simulink model "bustest2"  (R2018a)
settings: Solver=VariableStepAuto  StartTime=0.0  StopTime=10.0  RelTol=1e-3
undefined symbols (not defined in the file or in its folder): BandWidth, BaseVoltage, CogenEnabled, ControlledTransformerConnection, ControlledTransformerPowers, ControlledTransformerVoltages, ILDC, IsReversible, LDC_Z, m, MaxTap, MinTap, n, PTratio, RevBand, RevDelay, RevPowerThreshold, RevVreg, TapDelay, TapIncrement, TapLimitPerChange, TapWinding, UsingRegulatedBus, Vlimit, Vreg, VTerminal
settings Model: Creator=Michael Girbino  LastModifiedBy=Michael Girbino
settings CodeAppCC: StateflowObjectComments=on

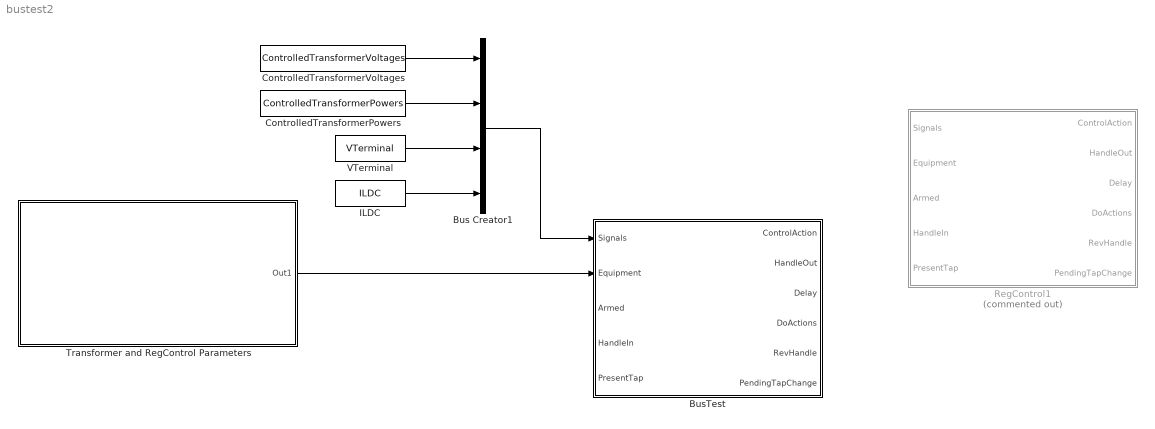
== system bustest2 ==
  Bus Creator1 : BusCreator  Inputs=4  OutDataTypeStr=Bus: SignalBus
  BusTest : Stateflow chart  TreatAsAtomicUnit=on
  ControlledTransformerPowers : Constant  Value=ControlledTransformerPowers
  ControlledTransformerVoltages : Constant  Value=ControlledTransformerVoltages
  ILDC : Constant  Value=ILDC
  RegControl1 : Stateflow chart  Commented=on  TreatAsAtomicUnit=on
  Transformer and RegControl Parameters : Subsystem
  VTerminal : Constant  Value=VTerminal
  wires:
  ControlledTransformerVoltages/1 -> Bus Creator1/1
  ControlledTransformerPowers/1 -> Bus Creator1/2
  Bus Creator1/1 -> BusTest/1(Signals)
  VTerminal/1 -> Bus Creator1/3
  ILDC/1 -> Bus Creator1/4
  Transformer and RegControl Parameters/1(Out1) -> BusTest/2(Equipment)

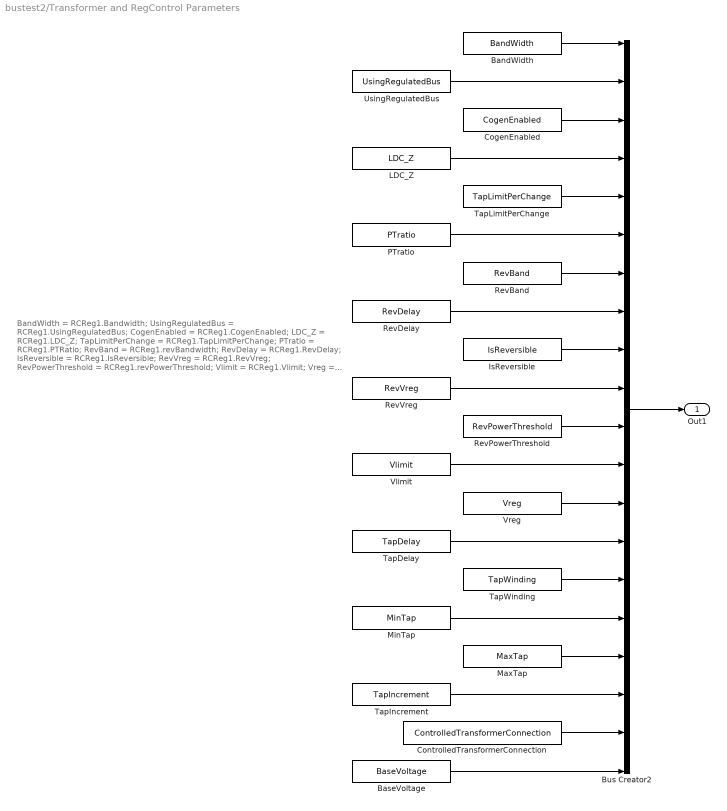
== system bustest2/Transformer and RegControl Parameters ==
  note: BandWidth = RCReg1.Bandwidth;
      | UsingRegulatedBus = RCReg1.UsingRegulatedBus;
      | CogenEnabled = RCReg1.CogenEnabled;
      | LDC_Z = RCReg1.LDC_Z;
      | TapLimitPerChange = RCReg1.TapLimitPerChange;
      | PTratio = RCReg1.PTRatio;
      | RevBand = RCReg1.revBandwidth;
      | RevDelay = RCReg1.RevDelay;
      | IsReversible = RCReg1.IsReversible;
      | RevVreg = RCReg1.RevVreg;
      | RevPowerThreshold = RCReg1.revPowerThreshold;
      | Vlimit = RCReg1.Vlimit;
      | Vreg = RCReg1.Vreg;
      | TapDelay = RCReg1.TapDelay;
      | TapWinding = RCReg1.xsfWinding;
      |
      | % PresentTap = Equipment.TReg1.Winding(TapWinding).puTap;
      | MinTap = TReg1.Winding(TapWinding).MinTap;
      | MaxTap = TReg1.Winding(TapWinding).MaxTap;
      | TapIncrement = TReg1.Winding(TapWinding).TapIncrement;
      | ControlledTransformerConnection = TReg1.Winding(TapWinding).Connection;
      | BaseVoltage = TReg1.Winding(TapWinding).Vbase;
  BandWidth : Constant  Value=BandWidth
  BaseVoltage : Constant  Value=BaseVoltage
  Bus Creator2 : BusCreator  Inputs=20  OutDataTypeStr=Bus: EquipmentBus
  CogenEnabled : Constant  Value=CogenEnabled
  ControlledTransformerConnection : Constant  Value=ControlledTransformerConnection
  IsReversible : Constant  Value=IsReversible
  LDC_Z : Constant  Value=LDC_Z
  MaxTap : Constant  Value=MaxTap
  MinTap : Constant  Value=MinTap
  PTratio : Constant  Value=PTratio
  RevBand : Constant  Value=RevBand
  RevDelay : Constant  Value=RevDelay
  RevPowerThreshold : Constant  Value=RevPowerThreshold
  RevVreg : Constant  Value=RevVreg
  TapDelay : Constant  Value=TapDelay
  TapIncrement : Constant  Value=TapIncrement
  TapLimitPerChange : Constant  Value=TapLimitPerChange
  TapWinding : Constant  Value=TapWinding
  UsingRegulatedBus : Constant  Value=UsingRegulatedBus
  Vlimit : Constant  Value=Vlimit
  Vreg : Constant  Value=Vreg
  Out1 : Outport
  wires:
  TapIncrement/1 -> Bus Creator2/18
  UsingRegulatedBus/1 -> Bus Creator2/2
  BandWidth/1 -> Bus Creator2/1
  BaseVoltage/1 -> Bus Creator2/20
  ControlledTransformerConnection/1 -> Bus Creator2/19
  MaxTap/1 -> Bus Creator2/17
  MinTap/1 -> Bus Creator2/16
  TapWinding/1 -> Bus Creator2/15
  TapDelay/1 -> Bus Creator2/14
  Vreg/1 -> Bus Creator2/13
  Vlimit/1 -> Bus Creator2/12
  RevPowerThreshold/1 -> Bus Creator2/11
  RevVreg/1 -> Bus Creator2/10
  IsReversible/1 -> Bus Creator2/9
  RevDelay/1 -> Bus Creator2/8
  RevBand/1 -> Bus Creator2/7
  PTratio/1 -> Bus Creator2/6
  TapLimitPerChange/1 -> Bus Creator2/5
  LDC_Z/1 -> Bus Creator2/4
  CogenEnabled/1 -> Bus Creator2/3
  Bus Creator2/1 -> Out1/1

== stateflow chart bustest2/RegControl1 ==
  settings: executeAtInitialization=1
  state ControlFlow
    state DetermineReversePendingLookingForward
      state CorrectFalseReversePending
        (default) -> (junction 108)
        (junction 108) -> (junction 109) [order 1] : [FwdPower < (-1*RevPowerThreshold)]
        (junction 108) -> (junction 111) [order 2]
        (junction 109) -> (junction 112) : {ReversePending = true;
            | RevHandle = ...
            | Push(ActionCodes.ACTION_REVERSE, ...
            | RevDelay);
            | }
        (junction 112) -> (junction 111)
      state CorrectTrueReversePending
        (default) -> (junction 804)
        (junction 804) -> (junction 123) [order 1] : [FwdPower >= (-1*RevPowerThreshold)]
        (junction 804) -> (junction 809) [order 2]
        (junction 123) -> (junction 806) : % Reset ReversePending:
            | % Delete RevHandle from ControlQueue
            | {DoActions.data = QueueActions.DELETE;
            | send(DoActions);
            | ReversePending = false;
            | RevHandle = 0;}
        (junction 806) -> (junction 809)
      state Finished
        en: GET_VOLTAGE = true;
      (default) -> (junction 106) : {FwdPower = -1*real( ControlledTransformerPower(ElementTerminal) );}
          | % Should we reverse?
      (junction 106) -> ControlFlow.DetermineReversePendingLookingForward.CorrectFalseReversePending [order 1] : [~ReversePending]
      (junction 106) -> (junction 110) [order 2]
      ControlFlow.DetermineReversePendingLookingForward.CorrectFalseReversePending -> (junction 110)
      (junction 110) -> (junction 120)
      (junction 120) -> ControlFlow.DetermineReversePendingLookingForward.CorrectTrueReversePending [order 1] : [ReversePending]
      (junction 120) -> (junction 122) [order 2]
      ControlFlow.DetermineReversePendingLookingForward.CorrectTrueReversePending -> (junction 122)
      (junction 122) -> ControlFlow.DetermineReversePendingLookingForward.Finished
    state DetermineReversePendingLookingReverseOrCogen
      state CorrectFalseReversePending
        (default) -> (junction 130)
        (junction 130) -> (junction 138) [order 1] : [FwdPower > RevPowerThreshold]
        (junction 130) -> (junction 137) [order 2]
        (junction 138) -> (junction 136) : {ReversePending = true;
            | RevHandle = ...
            | Push(ActionCodes.ACTION_REVERSE, ...
            | RevDelay);
            | }
        (junction 136) -> (junction 137)
      state CorrectTrueReversePending
        (default) -> (junction 154)
        (junction 154) -> (junction 799) [order 1] : [FwdPower <= RevPowerThreshold]
        (junction 154) -> (junction 792) [order 2]
        (junction 799) -> (junction 148) : % Reset ReversePending:
            | {ReversePending = false;}
        (junction 148) -> (junction 792)
      state Finished
        en: REV_NEUTRAL = true;
      (default) -> (junction 144) : {FwdPower = -1*real( ControlledTransformerPower(ElementTerminal) );}
          | % If reversed, check if power is back in forward direction
      (junction 144) -> ControlFlow.DetermineReversePendingLookingReverseOrCogen.CorrectFalseReversePending [order 1] : [~ReversePending]
      (junction 144) -> (junction 139) [order 2]
      ControlFlow.DetermineReversePendingLookingReverseOrCogen.CorrectFalseReversePending -> (junction 139)
      (junction 139) -> (junction 147)
      (junction 147) -> ControlFlow.DetermineReversePendingLookingReverseOrCogen.CorrectTrueReversePending [order 1] : [ReversePending]
      (junction 147) -> (junction 151) [order 2]
      ControlFlow.DetermineReversePendingLookingReverseOrCogen.CorrectTrueReversePending -> (junction 151)
      (junction 151) -> ControlFlow.DetermineReversePendingLookingReverseOrCogen.Finished
    state ReverseNeutralCase
      state Finished
        send(GET_VOLTAGE);
      state Exiting
        en: EXIT = true;
      (default) -> (junction 166)
      (junction 166) -> (junction 155) [order 1] : % tap change not specified as needed:
          | [~Armed]
      (junction 166) -> ControlFlow.ReverseNeutralCase.Finished [order 2]
      (junction 155) -> (junction 160) : {PendingTapChange = 0.0;}
      (junction 160) -> (junction 167) [order 1] : [abs(PresentTap - 1.0) < EPSILON]
      (junction 160) -> Exiting [order 2]
      (junction 167) -> (junction 518) : %{Increment = TapIncrement(TapWinding);
          | %PendingTapChange = round( (1.0 - ...
          | %PresentTap(TapWinding)) / Increment ) * Increment;}
          | {PendingTapChange = ...
          | round( (1.0 - TapWinding) / TapIncrement ) * TapIncrement;}
      (junction 518) -> (junction 519) [order 1] : [PendingTapChange ~= 0.0 && ~Armed]
      (junction 519) -> (junction 521) : {% Push ACTION_TAPCHANGE
          | % to ControlQueue with TapDelay:
          | Push(ActionCodes.ACTION_TAPCHANGE, TapDelay);
          | Armed = true;}
      (junction 518) -> (junction 520) [order 2]
      (junction 521) -> (junction 520)
      (junction 520) -> (junction 164)
      (junction 164) -> Exiting
    state GetVoltage
      state Finished
        en: DETERMINE_VLOCALBUS = true;
      (default) -> (junction 75)
      (junction 75) -> (junction 76) [order 1] : [UsingRegulatedBus]
      (junction 75) -> ControlFlow.GetVoltage.Finished [order 2] : {VBuffer = ControlledTransformerWindingVoltages;
          | %ControlledTransformer.GetWindingVoltages;
          | Vcontrol = GetControlVoltage;}
      (junction 76) -> (junction 78) : {TransformerConnection = ControlledTransformerConnection;
          | %TransformerConnection = ControlledTransformer.Winding(ElementTerminal).Connection;
          | %Vterminal = ComputeVTerminal;
          | }
      (junction 78) -> ControlFlow.GetVoltage.Finished
    state DetermineVlocalbus
      state Finished
        en: GET_VOLTAGEWLDC = true;
      (default) -> (junction 321)
      (junction 321) -> (junction 322) [order 1] : % Voltage limit for bus connected to regulated winding; default = 0.0 (inactive)
          | [VlimitActive]
      (junction 321) -> ControlFlow.DetermineVlocalbus.Finished [order 2] : {Vlocalbus = 0.0;}
      (junction 322) -> (junction 332)
      (junction 332) -> (junction 333) [order 1] : % when controlled transformer is different from LDC PTransformer
          | [UsingRegulatedBus]
      (junction 332) -> (junction 334) [order 2] : % controlled transformer is
          | % the LDC PTransformer
          | {Vlocalbus = abs(Vcontrol);}
      (junction 333) -> (junction 335) : {%ControlledTransformer.GetWindingVoltages(ElementTerminal, VBuffer);
          | Vlocalbus = abs( VBuffer(1) / PTRatio );}
      (junction 335) -> (junction 334)
      (junction 334) -> (junction 324)
      (junction 324) -> ControlFlow.DetermineVlocalbus.Finished
    state GetVoltageWithLDC
      state RX_LDCmode
        (default) -> (junction 365)
        (junction 365) -> (junction 366) [order 1] : [InReverseMode || InCogenMode]
        (junction 365) -> (junction 367) [order 2] : {VLDC = complex(R, X) * complex( real(ILDC), imag(ILDC) );}
        (junction 366) -> (junction 368) : {VLDC = complex(revR, revX) * complex( real(ILDC), imag(ILDC) );}
        (junction 368) -> (junction 367)
      state Z_LDCmode
        (default) -> (junction 387)
        (junction 387) -> (junction 388) [order 1] : [InReverseMode || InCogenMode]
        (junction 387) -> (junction 389) [order 2] : {Vcontrol = abs(Vcontrol) - abs(ILDC) * LDC_Z;}
        (junction 388) -> (junction 390) : {Vcontrol = abs(Vcontrol) - abs(ILDC) * revLDC_Z;}
        (junction 390) -> (junction 389)
      state Finished
        en: GET_TEST_VALUES = true;
      (default) -> (junction 354) : %{%%ControlledElement.GetCurrents(CBuffer);
          | %%Convert current to control current by CTRating:
          | %ILDC = ControlledElementCurrents( ControlledElementNconds * (ElementTerminal - 1) + ControlledPhase);}
      (junction 354) -> RX_LDCmode [order 1] : % Standard R, X LDC
          | [LDC_Z == 0.0]
      (junction 354) -> Z_LDCmode [order 2] : % Beckwith LDC_Z control mode
      Z_LDCmode -> ControlFlow.GetVoltageWithLDC.Finished
      RX_LDCmode -> ControlFlow.GetVoltageWithLDC.Finished
    state GetTestValues
      state Finished
        en:
        DETERMINE_TAP_CHANGE = true;
      (default) -> (junction 398) : % assumes looking forward:
          | {Vactual = abs(Vcontrol);}
      (junction 398) -> (junction 399) [order 1] : [InReverseMode]
      (junction 398) -> ControlFlow.GetTestValues.Finished [order 2] : {VregTest = Vreg;
          | BandTest = Bandwidth;}
      (junction 399) -> (junction 401) : {Vactual = Vactual / PresentTap;
          | VregTest = RevVreg;
          | BandTest = RevBandwidth;}
      (junction 401) -> ControlFlow.GetTestValues.Finished
    state DetermineTapChangeIsNeeded
      state Finished
        en:
        MAKE_TAP_CHANGE = true;
      (default) -> (junction 409)
      (junction 409) -> (junction 410) [order 1] : % difference between desired and actual > half bandwidth
          | [abs(VregTest - Vactual) > BandTest/2.0]
      (junction 409) -> ControlFlow.DetermineTapChangeIsNeeded.Finished [order 2] : {TapChangeIsNeeded = false;}
      (junction 410) -> (junction 412) : {TapChangeIsNeeded = true;}
      (junction 412) -> ControlFlow.DetermineTapChangeIsNeeded.Finished
    state MakeTapChange
      state GetVboostFromVlimit
        (default) -> (junction 441)
        (junction 441) -> (junction 446) [order 1] : [Vlocalbus > Vlimit]
        (junction 441) -> (junction 443) [order 2]
        (junction 446) -> (junction 445) : {Vboost = Vlimit - Vlocalbus;}
        (junction 445) -> (junction 443)
      state TapChangeUp
        (default) -> (junction 475)
        (junction 475) -> (junction 476) [order 1] : [PresentTap < MaxTap]
        (junction 475) -> (junction 477) [order 2]
        (junction 476) -> (junction 478) : {% push ACTION_TAPCHANGE to ControlQueue
            | % with delay ComputeTimeDelay(Vactual):
            | Push(ActionCodes.ACTION_TAPCHANGE, ...
            | ComputeTimeDelay(Vactual));
            | Armed = true;}
        (junction 478) -> (junction 477)
      state TapChangeDown
        (default) -> (junction 488) : % going down:
        (junction 488) -> (junction 489) [order 1] : [PresentTap > MinTap]
        (junction 488) -> (junction 490) [order 2]
        (junction 489) -> (junction 491) : {% push ACTION_TAPCHANGE to ControlQueue
            | % with delay ComputeTimeDelay(Vactual):
            | Push(ActionCodes.ACTION_TAPCHANGE, ...
            | ComputeTimeDelay(Vactual));
            | Armed = true;}
        (junction 491) -> (junction 490)
      state Finished
        en: FINISHED = true;
      (default) -> (junction 431) : % compute tapchange:
          | {Vboost = VregTest - Vactual;}
      (junction 431) -> (junction 432) [order 1] : [VlimitActive]
      (junction 431) -> (junction 433) [order 2]
      (junction 432) -> GetVboostFromVlimit
      GetVboostFromVlimit -> (junction 434)
      (junction 434) -> (junction 433)
      (junction 433) -> (junction 435) : {% PU winding boost needed:
          | BoostNeeded = Vboost * PTRatio / BaseVoltage;
          | Increment = TapIncrement(TapWinding);
          | % quantize to an increment:
          | PendingTapChange = round(BoostNeeded/Increment)*Increment;}
      (junction 435) -> (junction 453) : % send initial tap change message to ControlQueue, add delay time to solution control queue:
      (junction 453) -> (junction 454) [order 1] : % only changes 1 tap at a time:
          | [PendingTapChange ~= 0.0 && ~Armed]
      (junction 453) -> ControlFlow.MakeTapChange.Finished [order 2]
      (junction 454) -> (junction 464) : % see of any tap change is possible in desired direction (not saturated):
      (junction 464) -> TapChangeUp [order 1] : % going up:
          | [PendingTapChange > 0.0]
      (junction 464) -> TapChangeDown [order 2]
      TapChangeUp -> (junction 467)
      TapChangeDown -> (junction 466)
      (junction 467) -> (junction 466)
      (junction 466) -> (junction 456)
      (junction 456) -> ControlFlow.MakeTapChange.Finished
    state Finished
    (default) -> (junction 207) : {AssignInputsToLocals();
        | ResetTransitionFlags();}
    (junction 207) -> (junction 208) [order 2]
    (junction 208) -> (junction 86)
    (junction 207) -> (junction 529) [order 1] : [TapLimitPerChange == 0]
    (junction 86) -> (junction 87) [order 1] : [~UsingRegulatedBus]
    (junction 87) -> (junction 61)
    (junction 86) -> (junction 88) [order 2]
    (junction 61) -> (junction 62) [order 1] : [IsReversible || CogenEnabled]
    (junction 61) -> (junction 65) [order 2]
    (junction 62) -> (junction 63)
    (junction 63) -> DetermineReversePendingLookingForward [order 1] : [LookingForward && ~InCogenMode]
    (junction 63) -> DetermineReversePendingLookingReverseOrCogen [order 2]
    DetermineReversePendingLookingForward -> (junction 67) : [GET_VOLTAGE]
    DetermineReversePendingLookingReverseOrCogen -> (junction 175) : [REV_NEUTRAL]
    (junction 175) -> ReverseNeutralCase [order 1] : % mode for which tap change may be executed,
        | % but no reversal made:
        | [ReverseNeutral]
    (junction 175) -> (junction 174) [order 2]
    ReverseNeutralCase -> (junction 174) [order 2] : GET_VOLTAGE
    (junction 174) -> (junction 127)
    ReverseNeutralCase -> (junction 532) [order 1] : [EXIT]
    (junction 65) -> (junction 88)
    (junction 127) -> (junction 65)
    (junction 67) -> (junction 127)
    (junction 88) -> GetVoltage
    (junction 532) -> (junction 529)
    (junction 529) -> (junction 212)
    GetVoltage -> DetermineVlocalbus : [DETERMINE_VLOCALBUS]
    DetermineVlocalbus -> (junction 343) : [GET_VOLTAGEWLDC]
    (junction 343) -> GetVoltageWithLDC [order 1] : % line drop compensation, but not using regulated bus
        | [~UsingRegulatedBus && LDCActive]
    (junction 343) -> (junction 345) [order 2]
    GetVoltageWithLDC -> (junction 346) : [GET_TEST_VALUES]
    (junction 346) -> (junction 345)
    (junction 345) -> GetTestValues
    GetTestValues -> DetermineTapChangeIsNeeded : [DETERMINE_TAP_CHANGE]
    DetermineTapChangeIsNeeded -> (junction 420) : [MAKE_TAP_CHANGE]
    (junction 420) -> MakeTapChange [order 1] : [TapChangeIsNeeded]
    (junction 420) -> (junction 422) [order 2]
    MakeTapChange -> (junction 423) : [FINISHED]
    (junction 423) -> (junction 422)
    (junction 422) -> ControlFlow.Finished
    (junction 212) -> ControlFlow.Finished : {PendingTapChange = 0;}
  state h = Push(CodeVal, DelayVal) [function]
    (default) -> (junction 860) : {ActionCode = CodeVal;
        | Delay = DelayVal;
        | HandleOut = HandleOut + 1;
        | DoActions.data = QueueActions.PUSH;
        | send(DoActions);
        | h = HandleOut;}
  state AssignInputsToLocals [function]
    (default) -> (junction 987) : {BandWidth = Equipment.RCReg1.Bandwidth;
        | UsingRegulatedBus = Equipment.RCReg1.UsingRegulatedBus;
        | CogenEnabled = Equipment.RCReg1.CogenEnabled;
        | LDC_Z = Equipment.RCReg1.LDC_Z;
        | TapLimitPerChange = Equipment.RCReg1.TapLimitPerChange;
        | PTratio = Equipment.RCReg1.PTRatio;
        | RevBand = Equipment.RCReg1.revBandwidth;
        | RevDelay = Equipment.RCReg1.RevDelay;
        | IsReversible = Equipment.RCReg1.IsReversible;
        | RevVreg = Equipment.RCReg1.RevVreg;
        | RevPowerThreshold = Equipment.RCReg1.revPowerThreshold;
        | Vlimit = Equipment.RCReg1.Vlimit;
        | Vreg = Equipment.RCReg1.Vreg;
        | TapDelay = Equipment.RCReg1.TapDelay;
        | TapWinding = Equipment.RCReg1.xsfWinding;
        |
        | % PresentTap = Equipment.TReg1.Winding(TapWinding).puTap;
        | MinTap = Equipment.TReg1.Winding(TapWinding).MinTap;
        | MaxTap = Equipment.TReg1.Winding(TapWinding).MaxTap;
        | TapIncrement = Equipment.TReg1.Winding(TapWinding).TapIncrement;
        | ControlledTransformerConnection = Equipment.TReg1.Winding(TapWinding).Connection;
        | BaseVoltage = Equipment.TReg1.Winding(TapWinding).Vbase;
        |
        | ControlledTransformerWindingVoltages = Signals.ControlledTransformerWindingVoltages;
        | ControlledTransformerPower = Signals.ControlledTransformerPower;
        | VTerminal = Signals.VTerminal;
        | ILDC = Signals.ILDC;
        |
        | VBuffer = zeros(length(ControlledTransformerWindingVoltages));
        | }
    (junction 987) -> (junction 996) [order 1] : [Equipment.RCReg1.R~=0 || Equipment.RCReg1.X~=0 || Equipment.RCReg1.LDC_Z>0]
    (junction 987) -> (junction 991) [order 2] : {LDCActive = false;}
    (junction 996) -> (junction 990) : {LDCActive = true;}
    (junction 990) -> (junction 991)
    (junction 991) -> (junction 722)
    (junction 722) -> (junction 897) [order 1] : [HandleIn > HandleOut]
    (junction 722) -> (junction 898) [order 2]
    (junction 897) -> (junction 899) : {HandleOut = HandleIn;}
    (junction 899) -> (junction 898)
    (junction 898) -> (junction 900)
  note: BandWidth
      | UsingRegulatedBus
      | CogenEnabled
      | LDC_Z
      | TapLimitPerChange
      | PTratio
      | RevBand
      | IsReversible
      | RevVreg
      | Vlimit
      | Vreg
      | ILDC
      | FwdPower
  state ResetTransitionFlags [function]
    (default) -> (junction 886) : {DETERMINE_TAP_CHANGE = false;
        | DETERMINE_VLOCALBUS = false;
        | EXIT = false;
        | FINISHED = false;
        | GET_TEST_VALUES = false;
        | GET_VOLTAGE = false;
        | GET_VOLTAGEWLDC = false;
        | MAKE_TAP_CHANGE = false;
        | REV_NEUTRAL = false;}
  state UpdateControlledTransformerWV [function] [commented out]
    note: Retrieves new value for ControlledTransformerWindingVoltages. Update since last call of AssignInputsToLocals. Necessary because the control flow requires multiple updates to this quantity.
    (default) -> (junction 905) [commented out] : {ControlledTransformerWindingVoltages = ...
        | Inputs.ControlledTransformerWindingVoltages;}
  state UpdateControlledTransformerPower [function] [commented out]
    note: Retrieves new value for ControlledTransformerPower. Update since last call of AssignInputsToLocals. Necessary because the control flow requires multiple updates to this quantity.
    (default) -> (junction 902) [commented out] : {ControlledTransformerPower = ...
        | Inputs.ControlledTransformerPower;}
  state vt = ComputeVTerminal [function] [commented out]
    (default) -> (junction 309) [commented out] : % Iteration through order of admittance matrix
        | % (inherited from CktElement)
    (junction 310) -> (junction 308) [commented out] : [ii <= Yorder]
    (junction 308) -> (junction 311) [commented out] : {vt(ii) = NodeV(NodeRef(ii));}
    (junction 309) -> (junction 310) [commented out] : {ii = 1;}
    (junction 311) -> (junction 310) [commented out] : {ii = ii + 1;}
    (junction 310) -> (junction 312) [commented out]
  state WindingVoltages = GetWindingVoltages(Transformer, IndicatedWinding) [function] [commented out]
    note: Intend to store WindingVoltages in VBuffer.
        | Fills array with voltages across indicated winding
    note: For Delta connections or Line-Line voltages
    (default) -> (junction 969) [commented out] : % Determine whether winding exists
    (junction 923) -> (junction 921) [commented out] : [ii <= Yorder]
    (junction 921) -> (junction 924) [commented out] : {Vterminal(ii) = NodeV( NodeRef(i) );}
    (junction 969) -> (junction 922) [commented out] : [IndicatedWinding >= 1 && IndicatedWinding <= NumWindings]
    (junction 969) -> (junction 971) [commented out]
    (junction 922) -> (junction 923) [commented out] : {ii = 1;}
    (junction 924) -> (junction 923) [commented out] : {ii = ii + 1;}
    (junction 923) -> (junction 925) [commented out] : {k = (IndicatedWinding - 1) * Fnconds;
        | NeutTerm = Fnphases + k + 1;}
    (junction 925) -> (junction 935) [commented out] : {ii = 1;}
    (junction 935) -> (junction 933) [commented out] : [ii <= Fnphases]
    (junction 933) -> (junction 952) [commented out]
    (junction 952) -> (junction 953) [commented out] : [Winding(IndicatedWinding).Connection == Connections.WYE]
    (junction 952) -> (junction 956) [commented out]
    (junction 953) -> (junction 954) [commented out] : {VBuffer(ii) = Vterminal(ii + k) - Vterminal(NeutTerm);}
    (junction 954) -> (junction 955) [commented out]
    (junction 955) -> (junction 959) [commented out]
    (junction 956) -> (junction 957) [commented out] : [Winding(IndicatedWinding).Connection == Connections.DELTA]
    (junction 956) -> (junction 960) [commented out]
    (junction 957) -> (junction 958) [commented out] : {iii = RotatePhases(ii);
        | VBuffer(ii) = ...
        | Vterminal(ii + k) - ...
        | Vterminal(iii+k);}
    (junction 936) -> (junction 935) [commented out] : {ii = ii + 1;}
    (junction 935) -> (junction 937) [commented out] : {WindingVoltages = VBuffer;}
    (junction 958) -> (junction 959) [commented out]
    (junction 959) -> (junction 961) [commented out]
    (junction 961) -> (junction 960) [commented out]
    (junction 960) -> (junction 936) [commented out]
    (junction 937) -> (junction 971) [commented out]
    (junction 971) -> (junction 973) [commented out]
  state Result = GetControlVoltage [function]
    (default) -> (junction 236)
    (junction 236) -> (junction 237) [order 1] : [FPTphase == FPTphases.MAXPHASE]
        | % controlled phase is that with greatest |V|
    (junction 236) -> (junction 240) [order 2]
    (junction 237) -> (junction 260) : {ControlledPhase = 1;
        | % abs is equivalent to Cabs:
        | V = abs( VBuffer(ControlledPhase) );}
        | % Iteration through remaining phases:
    (junction 261) -> (junction 259) [order 1] : [ii <= Nphs]
    (junction 259) -> (junction 270)
    (junction 260) -> (junction 261) : {ii = 2;}
    (junction 270) -> (junction 271) [order 1] : [abs( VBuffer(ControlledPhase)) > V]
        | % if it's GREATER, make it the new V
    (junction 270) -> (junction 272) [order 2]
    (junction 271) -> (junction 273) : {V = VBuffer(ControlledPhase);
        | ControlledPhase = ii;}
    (junction 262) -> (junction 261) : {ii = ii+1;}
    (junction 261) -> (junction 238) [order 2]
    (junction 273) -> (junction 272)
    (junction 272) -> (junction 262) : {Result = VBuffer(FPTphase) / PTRatio;
        | % Complex divided by real
        | }
    (junction 238) -> (junction 239)
    (junction 239) -> (junction 243)
    (junction 240) -> (junction 241) [order 1] : [FPTphase == FPTphases.MINPHASE]
        | % controlled phase is that with least |V|
    (junction 241) -> (junction 282) : {ControlledPhase = 1;
        | % abs is equivalent to Cabs:
        | V = abs( VBuffer(ControlledPhase) );}
        | % Iteration through remaining phases:
    (junction 240) -> (junction 244) [order 2] : % just use one phase because
        | % that's what most controls do:
        | {Result = VBuffer(ControlledPhase) / PTRatio;
        | ControlledPhase = FPTphase;}
    (junction 278) -> (junction 277) [order 1] : [ii <= Nphs]
    (junction 277) -> (junction 291)
    (junction 282) -> (junction 278) : {ii = 2;}
    (junction 291) -> (junction 292) [order 1] : [abs( VBuffer(ControlledPhase)) < V]
        | % if it's LESS, make it the new V
    (junction 291) -> (junction 293) [order 2]
    (junction 292) -> (junction 294) : {V = VBuffer(ControlledPhase);
        | ControlledPhase = ii;}
    (junction 280) -> (junction 278) : {ii = ii+1;}
    (junction 278) -> (junction 242) [order 2]
    (junction 294) -> (junction 293)
    (junction 293) -> (junction 280) : {Result = VBuffer(FPTphase) / PTRatio;
        | % Complex divided by real
        | }
    (junction 242) -> (junction 243)
    (junction 243) -> (junction 245)
    (junction 245) -> (junction 244)
    (junction 244) -> (junction 246)
  state Result = ComputeTimeDelay(Vavg) [function]
    (default) -> (junction 507)
    (junction 507) -> (junction 508) [order 1] : [Finversetime]
    (junction 507) -> (junction 509) [order 2] : % determines which regulator control will act first,
        | % default is 15s
        | {Result = TimeDelay;}
    (junction 508) -> (junction 510) : % TimeDelay is adjusted inversely proportional to
        | % the amount that voltage is outside the band,
        | % down to 10 percent of specified time delay
        | % (Further out of band = band - 1> less time delay)
        | {Result = TimeDelay / min(10.0, 2.0*abs(Vreg - Vavg)/Bandwidth);}
    (junction 510) -> (junction 509)
    (junction 509) -> (junction 511)
  (default) -> ControlFlow
  data: CodeVal function_input; DelayVal function_input; h function_output; vt function_output; IndicatedPhase function_input; RotatedPhase function_output; Transformer function_input; IndicatedWinding function_input; WindingVoltages function_output; Result function_output; Vavg function_input; Result function_output; Signals input Bus: SignalBus; Equipment input Bus: EquipmentBus; BandTest local double =0; BoostNeeded local double =0; Increment local double =0; ReversePending local boolean =false; TapChangeIsNeeded local boolean =false; Vactual local double =0; Vboost local double =0; Vcontrol local double =0; Vlocalbus local double =0; VregTest local double =0; EPSILON local double =1.0e-12; R local double =0; X local double =0; BaseVoltage local double; ControlledPhase local uint8; ElementTerminal local uint8 =1; InCogenMode local boolean =false; InReverseMode local boolean =false; LDCActive local boolean =false; LookingForward local boolean =false; MaxTap local uint8; MinTap local uint8; NodeV local double; RevPowerThreshold local double; ReverseNeutral local boolean =false; TapIncrement local double; TapWinding local uint8 =1; VBuffer local double; VlimitActive local boolean =false; revLDC_Z local double =0; revR local double =0; revX local double =0; TransformerConnection local int32 =0; VLDC local double =0; Vterminal local double; Bandwidth local double =3; CogenEnabled local boolean =false; FwdPower local double =0; ILDC local double =0; IsReversible local boolean =false; LDC_Z local double =0; PTRatio local double =60; RevBandwidth local double =3; RevVreg local double =120; TapLimitPerChange local uint8 =16; UsingRegulatedBus local boolean =false; Vlimit local double =0; Vreg local double =120; ControlAction output Enum: ActionCodes; Armed input boolean =false; HandleOut output double =0; Delay output double =0; DoActions output Enum: QueueActions; RevBackHandle local uint8 =0; RevHandle output uint8 =0; REV_NEUTRAL local boolean =false; RevDelay local double; ControlledTransformerWindingVoltages local double; ControlledTransformerConnection local Enum: Connections; EXIT local boolean =false; FINISHED local boolean =false; GET_TEST_VALUES local boolean =false; MAKE_TAP_CHANGE local boolean =false; DETERMINE_TAP_CHANGE local boolean =false; GET_VOLTAGE local boolean =false; GET_VOLTAGEWLDC local boolean =false; DETERMINE_VLOCALBUS local boolean =false; TapDelay local double; HandleIn input double; PendingTapChange output double; PresentTap input double; ControlledElementCurrents local double; ControlledElementNconds local double; ControlledTransformerPower local double
  function RotatedPhase = RotatePhases(IndicatedPhase):
    | function RotatedPhase = RotatePhases(IndicatedPhase)
    |     HVLeadsLV = false;
    |     % FIRST NEED TO DETERMINE DELTADIRECTION:
    |     % If high voltage is delta, delta leads y (1)
    |     % If high voltage is wye, delta lags wye (2)
    |     if Winding(1).connection = Winding(2).connection
    |         DeltaDirection = 1;
    |     else
    |         if Winding(1).kvll >= Winding(2).kvll
    |             iHvolt = 1;
    |         else
    |             iHVolt = 2;
    |         end
    |         switch Winding(iHvolt).Connection
    |             case 0
    |                 if HVLeadsLV
    |                     DeltaDirection = -1;
    |                 else
    |                     DeltaDirection = 1;
    |                 end
    |             case 1
    |                 if HVLeadsLV
    |                     DeltaDirection = 1;
    |                 else
    |                     DeltaDirection = -1;
    |                 end
    |         end
    |     end
    |     
    |     % NOW, ACTUALLY DETERMINE PHASE ROTATION
    |     RotatedPhase = IndicatedPhase + DeltaDirection;
    | 
    |     % make sure RotatedPhase is within limits:
    |     if fNphases > 2
    |         % Assumes 2 phase delta is open delta
    |         if RotatedPhase > fNphases
    |             RotatedPhase = 1;
    |         elseif RotatedPhase < 1
    |             RotatedPhase = fNphases;
    |         end
    |     elseif RotatedPhase < 1
    |         RotatedPhase = 3; % For 2-phase delta, next phase will be 3rd phase
    |     end
    | end

== stateflow chart bustest2/BusTest ==
  settings: executeAtInitialization=1
  (default) -> (junction 997) : {BandWidth = Equipment.BandWidth;
      | UsingRegulatedBus = Equipment.UsingRegulatedBus;
      | CogenEnabled = Equipment.CogenEnabled;
      | LDC_Z = Equipment.LDC_Z;
      | TapLimitPerChange = Equipment.TapLimitPerChange;
      | PTratio = Equipment.PTratio;
      | RevBand = Equipment.RevBand;
      | RevDelay = Equipment.RevDelay;
      | IsReversible = Equipment.IsReversible;
      | RevVreg = Equipment.RevVreg;
      | RevPowerThreshold = Equipment.RevPowerThreshold;
      | Vlimit = Equipment.Vlimit;
      | Vreg = Equipment.Vreg;
      | TapDelay = Equipment.TapDelay;
      | TapWinding = Equipment.TapWinding;
      |
      | % PresentTap = Equipment.TReg1.Winding(TapWinding).puTap;
      | MinTap = Equipment.MinTap;
      | MaxTap = Equipment.MaxTap;
      | TapIncrement = Equipment.TapIncrement;
      | ControlledTransformerConnection = Equipment.ControlledTransformerConnection;
      | BaseVoltage = Equipment.BaseVoltage;
      |
      | ControlledTransformerWindingVoltages = Signals.ControlledTransformerVoltages;
      | ControlledTransformerPower = Signals.ControlledTransformerPowers;
      | VTerminal = Signals.VTerminal;
      | ILDC = Signals.ILDC;
      |
      | VBuffer = zeros(length(ControlledTransformerWindingVoltages));
      | }
  data: Signals input Bus: SignalBus; Equipment input Bus: EquipmentBus; BandTest local double =0; BoostNeeded local double =0; Increment local double =0; ReversePending local boolean =false; TapChangeIsNeeded local boolean =false; Vactual local double =0; Vboost local double =0; Vcontrol local double =complex(0); Vlocalbus local double =0; VregTest local double =0; EPSILON local double =1.0e-12; R local double =0; X local double =0; BaseVoltage local double =0; ControlledPhase local uint8; ElementTerminal local uint8 =uint8(1); InCogenMode local boolean =false; InReverseMode local boolean =false; LDCActive local boolean =false; LookingForward local boolean =false; MaxTap local double; MinTap local double; NodeV local double; RevPowerThreshold local double; ReverseNeutral local boolean =false; TapIncrement local double; TapWinding local uint8 =uint8(1); VBuffer local double; VlimitActive local boolean =false; revLDC_Z local double =0; revR local double =0; revX local double =0; TransformerConnection local uint8 =uint8(0); Vterminal local double; Bandwidth local double =3; CogenEnabled local boolean =false; FwdPower local double =0; ILDC local double =complex(0); IsReversible local boolean =false; LDC_Z local double =0; PTRatio local double =60; RevBandwidth local double =3; RevVreg local double =120; TapLimitPerChange local uint8 =uint8(16); UsingRegulatedBus local boolean =false; Vlimit local double =0; Vreg local double =120; ControlAction output Enum: ActionCodes; Armed input boolean =false; HandleOut output double =0; Delay output double =0; DoActions output Enum: QueueActions; RevBackHandle local uint8 =uint8(0); RevHandle output uint8 =uint8(0); REV_NEUTRAL local boolean =false; RevDelay local double; ControlledTransformerWindingVoltages local double; ControlledTransformerConnection local uint8; EXIT local boolean =false; FINISHED local boolean =false; GET_TEST_VALUES local boolean =false; MAKE_TAP_CHANGE local boolean =false; DETERMINE_TAP_CHANGE local boolean =false; GET_VOLTAGE local boolean =false; GET_VOLTAGEWLDC local boolean =false; DETERMINE_VLOCALBUS local boolean =false; TapDelay local double; HandleIn input double; PendingTapChange output double; PresentTap input double; ControlledElementCurrents local double; ControlledElementNconds local double; ControlledTransformerPower local double; BandWidth local; VTerminal local; PTratio local; RevBand local
